simulink model "PI_Controller"  (R2020a)
settings: Solver=VariableStepAuto  StartTime=0.0  StopTime=10.0  RelTol=1e-3
model workspace (MAT data in the model file):
  Ki = 41
  Kp = 310
values from neighbouring files (symbols this model uses):
  Ts = 0    [Data.mat]
settings Model: OrderedModelArguments=off  Creator=tanu  LastModifiedBy=tanu
settings DataIOCC: SaveOutput=off  SaveTime=off

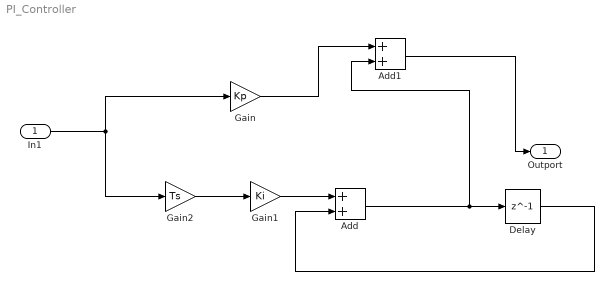
== system PI_Controller ==
  In1 : Inport  OutDataTypeStr=double  PortDimensions=1  SampleTime=0
  Add : Sum
  Add1 : Sum
  Delay : Delay  DelayLength=1
  Gain : Gain  Gain=Kp
  Gain1 : Gain  Gain=Ki
  Gain2 : Gain  Gain=Ts
  Outport : Outport
  wires:
  In1/1 -> Gain/1, Gain2/1
  Gain/1 -> Add1/1
  Gain2/1 -> Gain1/1
  Add1/1 -> Outport/1
  Gain1/1 -> Add/1
  Add/1 -> Add1/2, Delay/1
  Delay/1 -> Add/2
